simulink model "DC_motor_PIDcascade_c"  (R2015b)
settings: Solver=VariableStepAuto  StartTime=0.0  StopTime=10  MaxStep=1e-2  RelTol=1e-3
undefined symbols (not defined in the file): P_C
settings Model: Creator=mgreiff  LastModifiedBy=mgreiff
settings DebuggingCC: AlgebraicLoopMsg=none

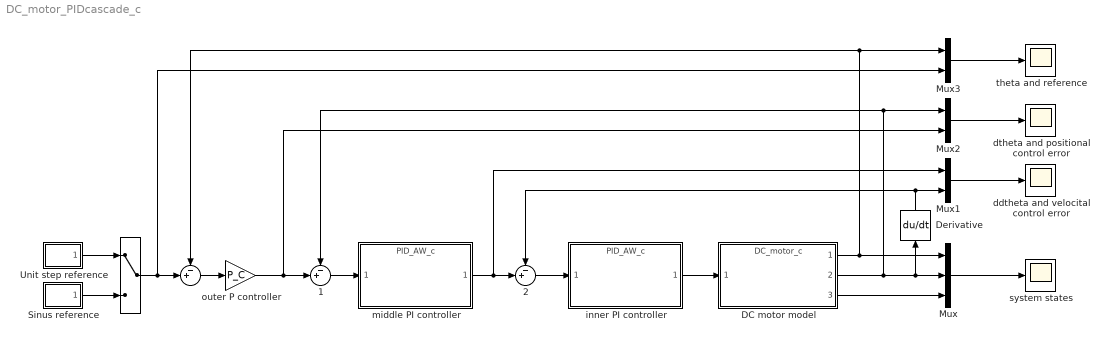
== system DC_motor_PIDcascade_c ==
  "   " : ManualSwitch
  "     " : Sum  Inputs=-+|
  " 1" : Sum  Inputs=-+|
  " 2" : Sum  Inputs=-+|
  DC motor model : ModelReference  ModelNameDialog=DC_motor_c.slx  SimulationMode=Normal  ModelReferenceVersion=1.7  CopyOfModelName=DC_motor_c.slx
  Derivative : Derivative
  Mux : Mux  Inputs=3
  Mux1 : Mux  Inputs=2
  Mux2 : Mux  Inputs=2
  Mux3 : Mux  Inputs=2
  Sinus reference : Subsystem
  Unit step reference : Subsystem
  ddtheta and velocital control error : Scope
  dtheta and positional control error : Scope
  "inner PI controller   " : ModelReference  ModelNameDialog=PID_AW_c.slx  SimulationMode=Normal  ModelReferenceVersion=1.4  CopyOfModelName=PID_AW_c.slx
  middle PI controller : ModelReference  ModelNameDialog=PID_AW_c.slx  SimulationMode=Normal  ModelReferenceVersion=1.4  CopyOfModelName=PID_AW_c.slx
  outer P controller : Gain  Gain=P_C
  system states : Scope
  theta and reference : Scope
  wires:
  DC motor model/1 -> Mux/1, Mux3/1, "     "/1
  DC motor model/3 -> Mux/3
  Mux/1 -> system states/1
  Unit step reference/1(voltage) -> "   "/1
  Sinus reference/1(voltage) -> "   "/2
  DC motor model/2 -> Derivative/1, Mux/2, " 1"/1, Mux2/1
  Mux2/1 -> dtheta and positional control error/1
  " 1"/1 -> middle PI controller/1
  outer P controller/1 -> " 1"/2, Mux2/2
  "     "/1 -> outer P controller/1
  Mux3/1 -> theta and reference/1
  "   "/1 -> Mux3/2, "     "/2
  " 2"/1 -> "inner PI controller   "/1
  "inner PI controller   "/1 -> DC motor model/1
  middle PI controller/1 -> Mux1/1, " 2"/2
  Mux1/1 -> ddtheta and velocital control error/1
  Derivative/1 -> " 2"/1, Mux1/2

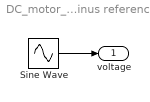
== system DC_motor_PIDcascade_c/Sinus reference ==
  Sine Wave : Sin  Frequency=2*pi/10  SampleTime=0
  voltage : Outport
  wires:
  Sine Wave/1 -> voltage/1

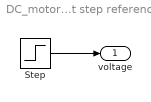
== system DC_motor_PIDcascade_c/Unit step reference ==
  Step : Step  SampleTime=0
  voltage : Outport
  wires:
  Step/1 -> voltage/1
